simulink model "GalvoPHD"  (Simulink 8.1)
settings: Solver=ode45  StartTime=0.0  StopTime=2  MaxStep=1e-3  MinStep=100e-6  RelTol=1e-3
settings Model: Creator=mainster  LastModifiedBy=mainster

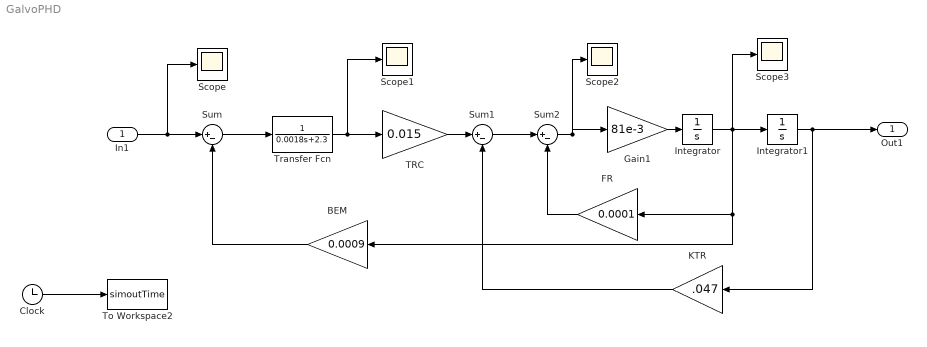
== system GalvoPHD ==
  In1 : Inport
  BEM : Gain  Gain=0.0009
  Clock : Clock
  FR : Gain  Gain=0.0001
  Gain1 : Gain  Gain=81e-3
  Integrator : Integrator
  Integrator1 : Integrator
  KTR : Gain  Gain=.047
  Scope{,1..3} (4 alike) : Scope
      Scope2 settings: SaveName=ScopeData2
      Scope3 settings: SaveName=ScopeData3
  Sum : Sum  Inputs=|+-
  Sum1 : Sum  Inputs=|+-
  Sum2 : Sum  Inputs=|+-
  TRC : Gain  Gain=0.015
  To Workspace2 : ToWorkspace  VariableName=simoutTime  SampleTime=-1  SaveFormat=Structure
  Transfer Fcn : TransferFcn  Denominator=[0.0018 2.3]
  Out1 : Outport
  wires:
  Clock/1 -> To Workspace2/1
  In1/1 -> Sum/1, Scope/1
  Sum/1 -> Transfer Fcn/1
  Transfer Fcn/1 -> TRC/1, Scope1/1
  TRC/1 -> Sum1/1
  Sum1/1 -> Sum2/1
  Sum2/1 -> Gain1/1, Scope2/1
  Gain1/1 -> Integrator/1
  Integrator/1 -> Integrator1/1, FR/1, BEM/1, Scope3/1
  Integrator1/1 -> Out1/1, KTR/1
  KTR/1 -> Sum1/2
  BEM/1 -> Sum/2
  FR/1 -> Sum2/2
